simulink model "Baseline"  (R2018a)
settings: Solver=FixedStepDiscrete  StartTime=0.0  StopTime=0.04  RelTol=1e-3
InitFcn:
  | Fs = 20e6;
  | res = 1;
  | SFDR = 100;
  | N = ceil(log2(Fs/res));
  | %trueRes = Fs/(2^N);
  | %phaseInc = round(Fc*2^N/Fs);
  | QAB = round((SFDR-12)/6);
  | Dither = N - QAB;
  | 
  | %% LLTF
  | a = load('lltf.mat');
  | lltfFlip = conj(flipud(a.LLTF(:, 1)));
  | 
  | lltfFlip = lltfFlip./(max(abs(lltfFlip))) .* 2^0;
libraries: dsphdlfiltering x2, commsource2 x1, dspbuff3 x1, dspmathops x1, dspsigops x1, commrflib2 x1
settings Model: DataTypeOverride=Off  SimulationMode=accelerator  Creator=tcollins  LastModifiedBy=tcollins
settings DataIOCC: LimitDataPoints=on  SaveOutput=off  SaveTime=off
settings OptimizationCC: BlockReduction=off  ConditionallyExecuteInputs=off  DefaultParameterBehavior=Inlined  LifeSpan=inf
settings DebuggingCC: AlgebraicLoopMsg=error  SingleTaskRateTransMsg=error  AllowSymbolicDim=off  StrictBusMsg=ErrorOnBusTreatedAsVector  SFUnexpectedBacktrackingDiag=warning  SFNoUnconditionalDefaultTransitionDiag=warning  SFExecutionAtInitializationDiag=none
settings HardwareCC: ProdBitPerPointer=32  ProdBitPerSizeT=32  ProdBitPerPtrDiffT=32  ProdLargestAtomicFloat=None  ProdIntDivRoundTo=Undefined  ProdEndianess=Unspecified  ProdWordSize=32  ProdHWDeviceType=ASIC/FPGA->ASIC/FPGA  ProdEqTarget=off
settings CodeAppCC: StateflowObjectComments=on
settings GRTTargetCC: TargetLangStandard=C89/C90 (ANSI)  GeneratePreprocessorConditionals=Disable all
settings ConfigComp: CovScope=ReferencedModels  CovMetricSettings=dw  CovHtmlReporting=on  CovSaveCumulativeToWorkspaceVar=on  CovSaveSingleToWorkspaceVar=on  CovExternalEMLEnable=off  CovSFcnEnable=off

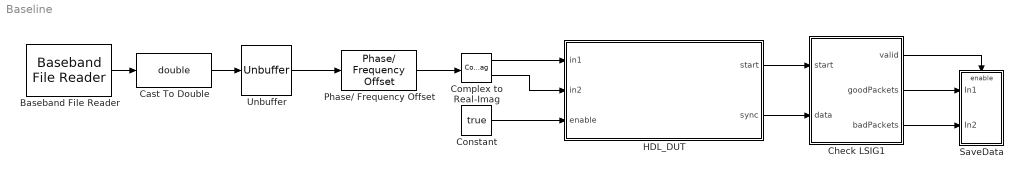
== system Baseline ==
  Baseband File Reader : commsource2/Baseband File Reader  Filename=BeaconsLoopbackInt16.bb  InheritSampleTimeFromFile=on  SampleTime=1  SamplesPerFrame=2500  CyclicRepetition=off  FileEndOutputPort=off  SimulateUsing=Code generation
      settings: SourceProductName=Communications System Toolbox  SourceProductBaseCode=CM
  Cast To Double : DataTypeConversion  OutDataTypeStr=double
  Check LSIG1 : MATLAB Function  TreatAsAtomicUnit=on
  Complex to Real-Imag : ComplexToRealImag
  Constant : Constant  Value=true  SampleTime=-1
  HDL_DUT : Subsystem
  Phase/ Frequency Offset : commrflib2/Phase// Frequency Offset  phaseOffset=0  freqPort=off  freqOffset=0
      settings: SourceProductName=Communications System Toolbox
  SaveData : Subsystem
  Unbuffer : Unbuffer
  wires:
  Complex to Real-Imag/1 -> HDL_DUT/1(in1)
  Complex to Real-Imag/2 -> HDL_DUT/2(in2)
  Unbuffer/1 -> Phase/ Frequency Offset/1
  Baseband File Reader/1 -> Cast To Double/1
  Cast To Double/1 -> Unbuffer/1
  HDL_DUT/2(sync) -> Check LSIG1/2(data)
  HDL_DUT/1(start) -> Check LSIG1/1(start)
  Check LSIG1/3(badPackets) -> SaveData/2(In2)
  Check LSIG1/2(goodPackets) -> SaveData/1(In1)
  Check LSIG1/1(valid) -> SaveData/Enable
  Constant/1 -> HDL_DUT/3(enable)
  Phase/ Frequency Offset/1 -> Complex to Real-Imag/1

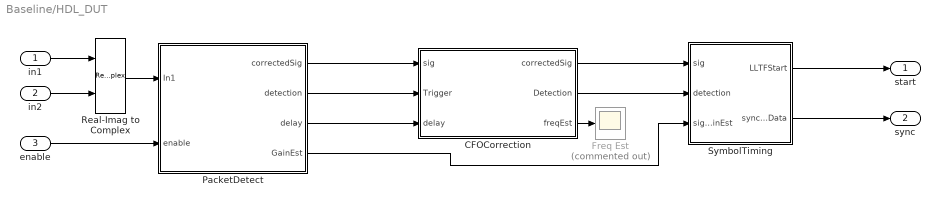
== system Baseline/HDL_DUT ==
  in1 : Inport
  in2 : Inport  Port=2
  enable : Inport  Port=3
  CFOCorrection : Subsystem
  Freq Est : Scope  Commented=on
  PacketDetect : Subsystem
  Real-Imag to Complex : RealImagToComplex
  SymbolTiming : Subsystem
  start : Outport
  sync : Outport  Port=2
  wires:
  in1/1 -> Real-Imag to Complex/1
  in2/1 -> Real-Imag to Complex/2
  Real-Imag to Complex/1 -> PacketDetect/1(In1)
  CFOCorrection/3(freqEst) -> Freq Est/1
  PacketDetect/2(detection) -> CFOCorrection/2(Trigger)
  PacketDetect/4(GainEst) -> SymbolTiming/3(sigGainEst)
  SymbolTiming/1(LLTFStart) -> start/1
  SymbolTiming/2(syncedData) -> sync/1
  PacketDetect/3(delay) -> CFOCorrection/3(delay)
  PacketDetect/1(correctedSig) -> CFOCorrection/1(sig)
  CFOCorrection/1(correctedSig) -> SymbolTiming/1(sig)
  CFOCorrection/2(Detection) -> SymbolTiming/2(detection)
  enable/1 -> PacketDetect/2(enable)

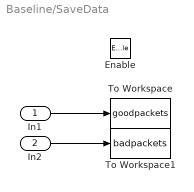
== system Baseline/SaveData ==
  In1 : Inport
  In2 : Inport  Port=2
  Enable : EnablePort
  To Workspace : ToWorkspace  VariableName=goodpackets  SampleTime=-1
      settings: Save2DSignal=2-D array (concatenate along first dimension)
  To Workspace1 : ToWorkspace  VariableName=badpackets  SampleTime=-1
      settings: Save2DSignal=2-D array (concatenate along first dimension)
  wires:
  In1/1 -> To Workspace/1
  In2/1 -> To Workspace1/1

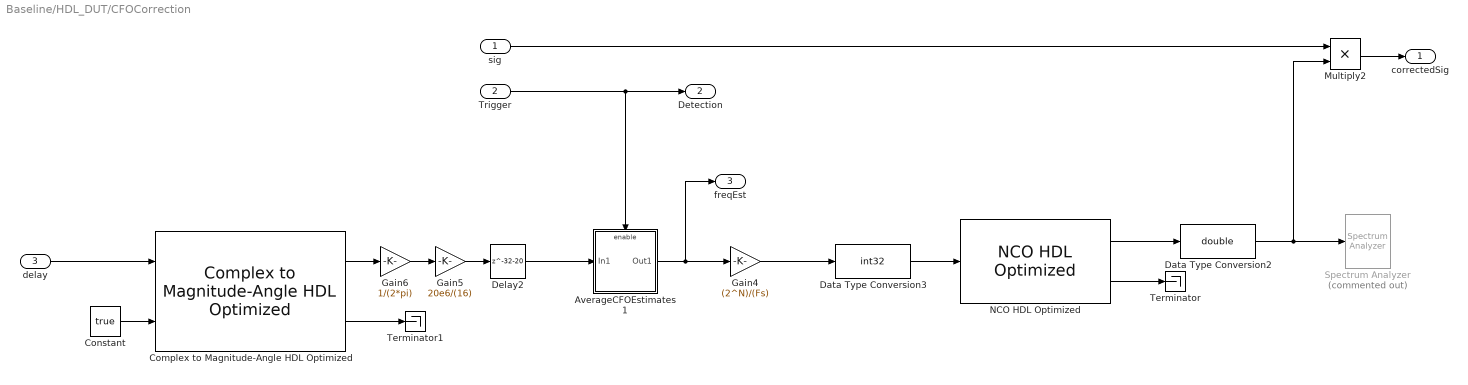
== system Baseline/HDL_DUT/CFOCorrection ==
  sig : Inport
  Trigger : Inport  Port=2
  delay : Inport  Port=3
  AverageCFOEstimates1 : Subsystem
  Complex to Magnitude-Angle HDL Optimized : dspmathops/Complex to Magnitude-Angle HDL Optimized  NumIterationsSource=Auto  NumIterations=10  OutputFormat=Angle  AngleFormat=Radians  ScaleOutput=on  SimulateUsing=Code generation
      settings: SourceProductName=DSP System Toolbox  SourceProductBaseCode=DS
  Constant : Constant  Value=true  SampleTime=-1
  Data Type Conversion2 : DataTypeConversion  OutDataTypeStr=double
  Data Type Conversion3 : DataTypeConversion  OutDataTypeStr=int32
  Delay2 : Delay  DelayLength=32-20
  Gain4 : Gain  Gain=(2^N)/(Fs)
  Gain5 : Gain  Gain=20e6/(16)
  Gain6 : Gain  Gain=1/(2*pi)
  Multiply2 : Product
  NCO HDL Optimized : dspsigops/NCO HDL Optimized  PhaseIncrementSource=Input port  PhaseIncrement=100  PhaseOffsetSource=Property  PhaseOffset=0  DitherSource=Property  NumDitherBits=Dither  PhaseQuantization=on  NumQuantizerAccumulatorBits=QAB  LUTCompress=off  ResetAction=off  ValidInputPort=off  Waveform=Complex exponential  PhasePort=off  SimulateUsing=Code generation  AccumulatorWL=N  OutputDataType=Binary point scaling  OutputWL=N-1  OutputFL=N-2
      settings: SourceProductName=DSP System Toolbox  SourceProductBaseCode=DS
  Spectrum Analyzer : SpectrumAnalyzer  Commented=on
  Terminator : Terminator
  Terminator1 : Terminator
  correctedSig : Outport
  Detection : Outport  Port=2
  freqEst : Outport  Port=3
  wires:
  Trigger/1 -> AverageCFOEstimates1/Enable, Detection/1
  delay/1 -> Complex to Magnitude-Angle HDL Optimized/1
  sig/1 -> Multiply2/1
  Multiply2/1 -> correctedSig/1
  Complex to Magnitude-Angle HDL Optimized/1 -> Gain6/1
  NCO HDL Optimized/1 -> Data Type Conversion2/1
  Data Type Conversion2/1 -> Spectrum Analyzer/1, Multiply2/2
  Gain4/1 -> Data Type Conversion3/1
  Delay2/1 -> AverageCFOEstimates1/1(In1)
  AverageCFOEstimates1/1(Out1) -> freqEst/1, Gain4/1
  Gain5/1 -> Delay2/1
  NCO HDL Optimized/2 -> Terminator/1
  Constant/1 -> Complex to Magnitude-Angle HDL Optimized/2
  Gain6/1 -> Gain5/1
  Data Type Conversion3/1 -> NCO HDL Optimized/1
  Complex to Magnitude-Angle HDL Optimized/2 -> Terminator1/1

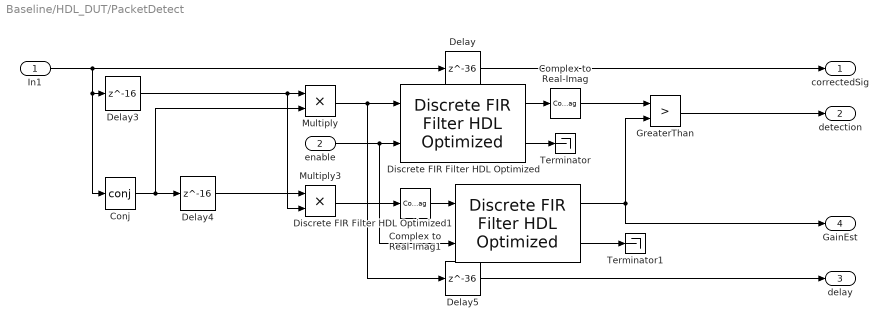
== system Baseline/HDL_DUT/PacketDetect ==
  In1 : Inport
  enable : Inport  Port=2
  Complex to Real-Imag : ComplexToRealImag  Output=Real
  Complex to Real-Imag1 : ComplexToRealImag  Output=Real
  Conj : Math  Operator=conj  SaturateOnIntegerOverflow=on
  Delay : Delay  DelayLength=36
  Delay3 : Delay  DelayLength=16
  Delay4 : Delay  DelayLength=16
  Delay5 : Delay  DelayLength=36
  Discrete FIR Filter HDL Optimized : dsphdlfiltering/Discrete FIR Filter HDL Optimized  Numerator=ones(1,16)  Sharing=off  SharingFactor=2  SimulateUsing=Code generation  roundingMode=Floor  overflowMode=on  CoefficientsDataTypeStr=Inherit: Same word length as input  CoefficientsMin=[]  CoefficientsMax=[]  OutputDataTypeStr=Inherit: Same word length as input  OutputMin=[]  OutputMax=[]  ValidInPort=on  ReadyPort=off
      settings: SourceProductName=DSP System Toolbox  SourceProductBaseCode=DS
  Discrete FIR Filter HDL Optimized1 : dsphdlfiltering/Discrete FIR Filter HDL Optimized  Numerator=ones(1,16)*0.7  Sharing=off  SharingFactor=2  SimulateUsing=Code generation  roundingMode=Floor  overflowMode=on  CoefficientsDataTypeStr=Inherit: Same word length as input  CoefficientsMin=[]  CoefficientsMax=[]  OutputDataTypeStr=Inherit: Same word length as input  OutputMin=[]  OutputMax=[]  ValidInPort=on  ReadyPort=off
      settings: SourceProductName=DSP System Toolbox  SourceProductBaseCode=DS
  GreaterThan : RelationalOperator  Operator=>  OutDataTypeStr=boolean  RndMeth=Simplest
  Multiply : Product
  Multiply3 : Product
  Terminator : Terminator
  Terminator1 : Terminator
  correctedSig : Outport
  detection : Outport  Port=2
  delay : Outport  Port=3
  GainEst : Outport  Port=4
  wires:
  Discrete FIR Filter HDL Optimized/1 -> Complex to Real-Imag/1
  In1/1 -> Delay/1, Delay3/1, Conj/1
  Conj/1 -> Multiply/2, Delay4/1
  GreaterThan/1 -> detection/1
  Complex to Real-Imag/1 -> GreaterThan/1
  Discrete FIR Filter HDL Optimized1/1 -> GainEst/1, GreaterThan/2
  Delay3/1 -> Multiply3/2, Multiply/1
  Multiply3/1 -> Complex to Real-Imag1/1
  Delay4/1 -> Multiply3/1
  Complex to Real-Imag1/1 -> Discrete FIR Filter HDL Optimized1/1
  Multiply/1 -> Discrete FIR Filter HDL Optimized/1, Delay5/1
  Discrete FIR Filter HDL Optimized/2 -> Terminator/1
  Discrete FIR Filter HDL Optimized1/2 -> Terminator1/1
  enable/1 -> Discrete FIR Filter HDL Optimized/2, Discrete FIR Filter HDL Optimized1/2
  Delay/1 -> correctedSig/1
  Delay5/1 -> delay/1

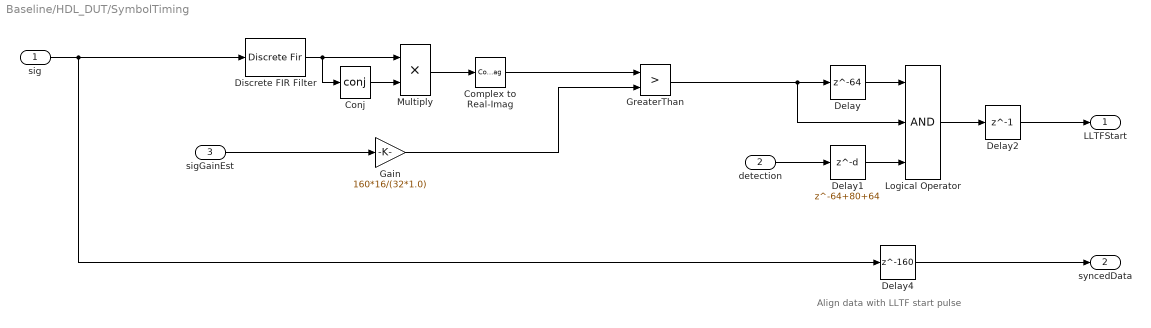
== system Baseline/HDL_DUT/SymbolTiming ==
  note: Align data with LLTF start pulse
  sig : Inport
  detection : Inport  Port=2
  sigGainEst : Inport  Port=3
  Complex to Real-Imag : ComplexToRealImag  Output=Real
  Conj : Math  Operator=conj  SaturateOnIntegerOverflow=on
  Delay : Delay  DelayLength=64
  Delay1 : Delay  DelayLength=64+80+64
  Delay2 : Delay  DelayLength=1
  Delay4 : Delay  DelayLength=160
  Discrete FIR Filter : DiscreteFir  Coefficients=lltfFlip(1:80).'
  Gain : Gain  Gain=160*16/(32*1.0)
  GreaterThan : RelationalOperator  Operator=>  OutDataTypeStr=boolean  RndMeth=Simplest
  Logical Operator : Logic  Inputs=3  AllPortsSameDT=off  OutDataTypeStr=boolean
  Multiply : Product
  LLTFStart : Outport
  syncedData : Outport  Port=2
  wires:
  Discrete FIR Filter/1 -> Conj/1, Multiply/1
  GreaterThan/1 -> Logical Operator/2, Delay/1
  Delay/1 -> Logical Operator/1
  sigGainEst/1 -> Gain/1
  detection/1 -> Delay1/1
  Multiply/1 -> Complex to Real-Imag/1
  Delay1/1 -> Logical Operator/3
  Logical Operator/1 -> Delay2/1
  Delay2/1 -> LLTFStart/1
  Conj/1 -> Multiply/2
  Complex to Real-Imag/1 -> GreaterThan/1
  Gain/1 -> GreaterThan/2
  sig/1 -> Discrete FIR Filter/1, Delay4/1
  Delay4/1 -> syncedData/1

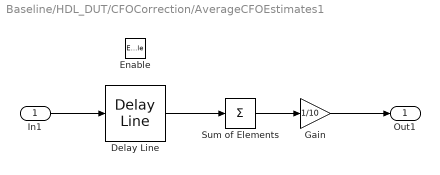
== system Baseline/HDL_DUT/CFOCorrection/AverageCFOEstimates1 ==
  In1 : Inport
  Enable : EnablePort
  Delay Line : dspbuff3/Delay Line  siz=10  ic=0  directfeed=off  enable_output=off  hold_output=off  OutputFrames=off
      settings: SourceProductName=DSP System Toolbox  SourceProductBaseCode=DS
  Gain : Gain  Gain=1/10
  Sum of Elements : Sum  Inputs=+
  Out1 : Outport
  wires:
  Delay Line/1 -> Sum of Elements/1
  In1/1 -> Delay Line/1
  Sum of Elements/1 -> Gain/1
  Gain/1 -> Out1/1

== matlab function Baseline/Check LSIG1 ==
  data: start input; data input; valid output; goodPackets output; badPackets output
function [valid,goodPackets,badPackets] = fcn(start,data)
%#codegen
% coder.extrinsic('offline');

persistent buff counter cfgRec largerCount chanEst noiseVar cfgNonHT numDataSym
persistent goodPacketsCount badPacketsCount
N = 160+80; 
M = 1e6;

if isempty(buff)
    buff = complex(zeros(M,1));
    counter = int16(N+1);
    cfgRec = wlanRecoveryConfig('EqualizationMethod', 'ZF');
    largerCount = 0;
    cfgNonHT = wlanNonHTConfig;
    numDataSym = 0;
    chanEst = 0;
    noiseVar = 0;
    goodPacketsCount = 0;
    badPacketsCount = 0;
end

valid = false;

if start
    counter = int16(1);
elseif counter <= N
    counter = counter + int16(1);
end

if counter<N
    buff(counter) = data;
end

if counter == N
    rxLLTF = buff(1:160);
    rxLSIG = buff(161:160+80);
    chanBW = 'CBW20';
    % Perform channel estimation based on L-LTF
    demodLLTF = wlanLLTFDemodulate(rxLLTF, chanBW, 1);
    noiseVar = helperNoiseEstimate(demodLLTF);
    chanEst = wlanLLTFChannelEstimate(demodLLTF, chanBW);
    % Recover information bits in L-SIG
    [recLSIGBits,failParityCheck] = wlanLSIGRecover(rxLSIG, chanEst, noiseVar, chanBW);
    if ~failParityCheck %isequal(ref,recLSIGBits.')
        rate = bi2de(double(recLSIGBits(1:3).'), 'left-msb');
        if rate <= 1
            cfgNonHT.MCS = rate + 6;
        else
            cfgNonHT.MCS = mod(rate, 6);
        end
        cfgNonHT.PSDULength = bi2de(double(recLSIGBits(6:17)'));
        largerCount = 1;
        numDataSym = offline(cfgNonHT);
    else
        fprintf('LSIG Invalid\n');
        badPacketsCount = badPacketsCount + 1;
    end
end

if largerCount > 0
    buff(largerCount) = data;
    largerCount = largerCount + 1;
    if largerCount > 80*numDataSym
        % Recover payload bits
        recBits = wlanNonHTDataRecover(buff(2:80*numDataSym+1), chanEst, ...
            noiseVar, cfgNonHT, cfgRec);        
        % Evaluate recovered bits
        [validBeacon, MPDU] = nonHTBeaconRxMPDUDecode(recBits);
        if validBeacon
            goodPacketsCount = goodPacketsCount + 1;
            nonHTBeaconRxOutputDisplay(MPDU); % Display SSID
            fprintf('Good packets captured: %d\n',int16(goodPacketsCount));
        else
            badPacketsCount = badPacketsCount + 1;
%             fprintf('Bad packets captured: %d\n',int16(badPacketsCount));
        end
        largerCount = 0;
        valid = true;
    end
end

goodPackets = goodPacketsCount;
badPackets = badPacketsCount;

end
